simulink model "switchcase"  (Simulink 6.6)
settings: Solver=ode3  StartTime=0.0  StopTime=10.0  FixedStep=1  RelTol=1e-3
settings Model: Creator=hnine  LastModifiedBy=hnine

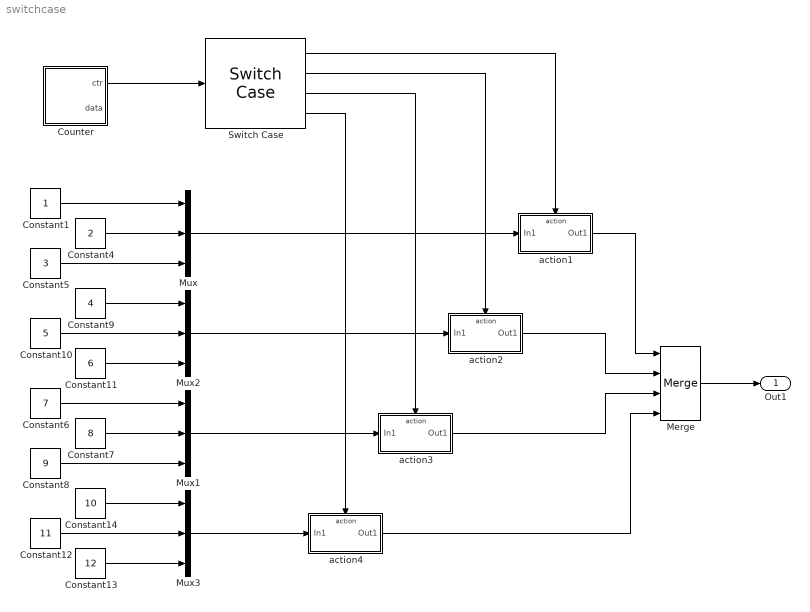
== system switchcase ==
  Constant1 : Constant
  Constant10 : Constant  Value=5
  Constant11 : Constant  Value=6
  Constant12 : Constant  Value=11
  Constant13 : Constant  Value=12
  Constant14 : Constant  Value=10
  Constant4 : Constant  Value=2
  Constant5 : Constant  Value=3
  Constant6 : Constant  Value=7
  Constant7 : Constant  Value=8
  Constant8 : Constant  Value=9
  Constant9 : Constant  Value=4
  Counter : Stateflow chart
  Merge : Merge  Inputs=4
  Mux{,1..3} (4 alike) : Mux  Inputs=3
  Switch Case : SwitchCase  CaseConditions={1,[2,3],4}
  action1 : Subsystem  TreatAsAtomicUnit=on
  action2 : Subsystem  TreatAsAtomicUnit=on
  action3 : Subsystem  TreatAsAtomicUnit=on
  action4 : Subsystem  TreatAsAtomicUnit=on
  Out1 : Outport
  wires:
  Switch Case/1 -> action1/Action
  Switch Case/2 -> action2/Action
  Switch Case/3 -> action3/Action
  Switch Case/4 -> action4/Action
  action1/1(Out1) -> Merge/1
  action2/1(Out1) -> Merge/2
  action3/1(Out1) -> Merge/3
  action4/1(Out1) -> Merge/4
  Merge/1 -> Out1/1
  Constant1/1 -> Mux/1
  Constant4/1 -> Mux/2
  Constant5/1 -> Mux/3
  Mux/1 -> action1/1(In1)
  Constant6/1 -> Mux1/1
  Constant7/1 -> Mux1/2
  Constant8/1 -> Mux1/3
  Constant9/1 -> Mux2/1
  Constant10/1 -> Mux2/2
  Constant11/1 -> Mux2/3
  Constant14/1 -> Mux3/1
  Constant12/1 -> Mux3/2
  Constant13/1 -> Mux3/3
  Mux2/1 -> action2/1(In1)
  Mux1/1 -> action3/1(In1)
  Mux3/1 -> action4/1(In1)
  Counter/1(ctr) -> Switch Case/1

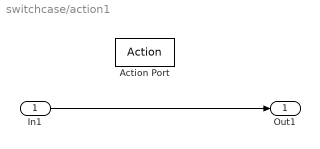
== system switchcase/action1 ==
  In1 : Inport
  Action Port : ActionPort  ActionType=case
  Out1 : Outport
  wires:
  In1/1 -> Out1/1

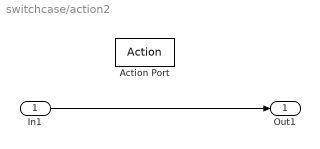
== system switchcase/action2 ==
  In1 : Inport
  Action Port : ActionPort  ActionType=case
  Out1 : Outport
  wires:
  In1/1 -> Out1/1

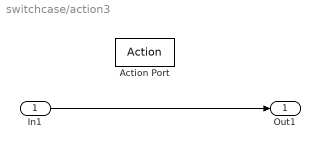
== system switchcase/action3 ==
  In1 : Inport
  Action Port : ActionPort  ActionType=case
  Out1 : Outport
  wires:
  In1/1 -> Out1/1

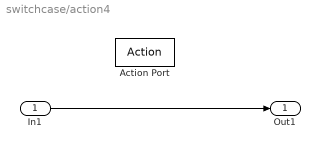
== system switchcase/action4 ==
  In1 : Inport
  Action Port : ActionPort  ActionType=default
  Out1 : Outport
  wires:
  In1/1 -> Out1/1

== stateflow chart Counter ==
  settings: executeAtInitialization=1
  state s1
  (default) -> s1
  s1 -> s1 [order 1] : [ctr < 3] / ctr = ctr+1;
  s1 -> s1 [order 2] : [ctr >= 3] / ctr = 1;
  data: ctr output double =1; data output double =-1
